simulink library "bsg"  (Simulink 8.1)
settings: Solver=ode1  StartTime=0.0  StopTime=Inf  FixedStep=0.001  RelTol=1e-3
PostLoadFcn:
  | , if any(exist('dsrtsu_mdlpostloadfcn', 'file') == [2, 3, 6]), try dsrtsu_mdlpostloadfcn('Execute', bdroot); catch fprintf('Error in PostLoadFcn (dsrtsu_mdlpostloadfcn) for model "%s":\n %s\n', bdroot, lasterr); end, end,
undefined symbols (not defined in the file or in its folder): KACC_ConsideredDistControlSetTimeGap_s, KACC_GapControlDesDistMarg_m, KACC_GapControlTGapPerc_perc, KACC_SteadyTGapPTBFixedMargin_flg
settings Model: DSRTSU_INTERNAL_RTI_VER=450  DSRTSU_INTERNAL_RTI_TYPE=rti1401  Creator=AT015555  LastModifiedBy=AT015555

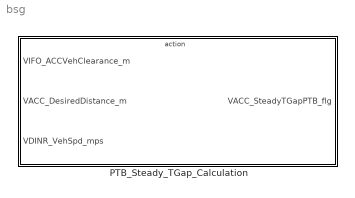
== system bsg ==
  PTB_Steady_TGap_Calculation : Subsystem  TreatAsAtomicUnit=on

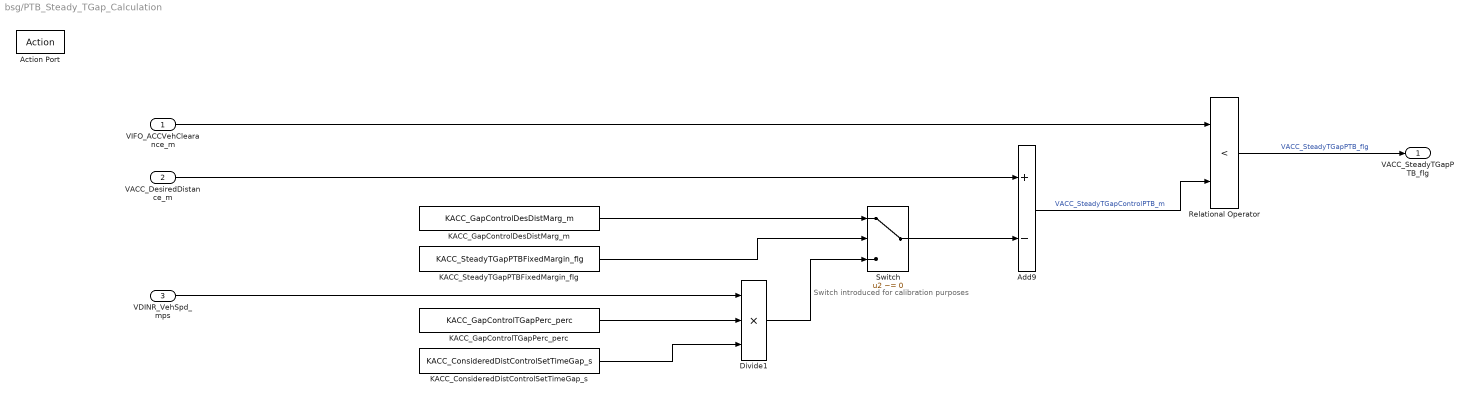
== system bsg/PTB_Steady_TGap_Calculation ==
  note: Switch introduced for calibration purposes
  VIFO_ACCVehClearance_m : Inport
  VACC_DesiredDistance_m : Inport  Port=2
  VDINR_VehSpd_mps : Inport  Port=3
  Action Port : ActionPort
  Add9 : Sum  Inputs=+-
  Divide1 : Product  Inputs=***
  KACC_ConsideredDistControlSetTimeGap_s : Constant  Value=KACC_ConsideredDistControlSetTimeGap_s
  KACC_GapControlDesDistMarg_m : Constant  Value=KACC_GapControlDesDistMarg_m
  KACC_GapControlTGapPerc_perc : Constant  Value=KACC_GapControlTGapPerc_perc
  KACC_SteadyTGapPTBFixedMargin_flg : Constant  Value=KACC_SteadyTGapPTBFixedMargin_flg
  Relational Operator : RelationalOperator  Operator=<  OutDataTypeStr=boolean
  Switch : Switch  Criteria=u2 ~= 0
  VACC_SteadyTGapPTB_flg : Outport
  wires:
  Add9/1 -> Relational Operator/2  "VACC_SteadyTGapControlPTB_m"
  VIFO_ACCVehClearance_m/1 -> Relational Operator/1
  VACC_DesiredDistance_m/1 -> Add9/1
  Relational Operator/1 -> VACC_SteadyTGapPTB_flg/1  "VACC_SteadyTGapPTB_flg"
  Switch/1 -> Add9/2
  KACC_SteadyTGapPTBFixedMargin_flg/1 -> Switch/2
  KACC_ConsideredDistControlSetTimeGap_s/1 -> Divide1/3
  KACC_GapControlTGapPerc_perc/1 -> Divide1/2
  VDINR_VehSpd_mps/1 -> Divide1/1
  Divide1/1 -> Switch/3
  KACC_GapControlDesDistMarg_m/1 -> Switch/1
